simulink subsystem "h_bridge_v2"  (R2023a)
settings: Solver=VariableStepAuto  StartTime=0.0  StopTime=10.0  RelTol=1e-3
libraries: fl_lib x7, nesl_utility x4, dspstat3 x1
settings Model: Creator=motya  LastModifiedBy=motya

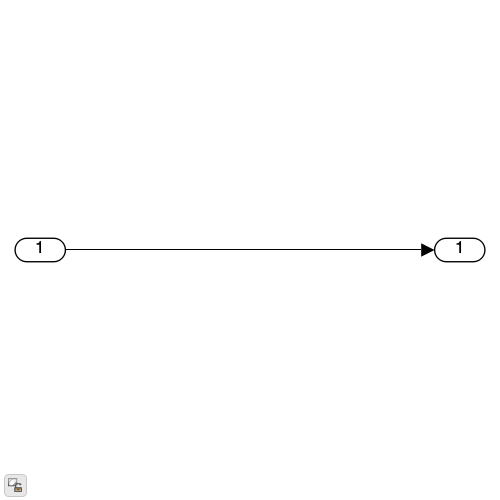
[thumbnail: Simulink's stored preview of the top-level diagram]
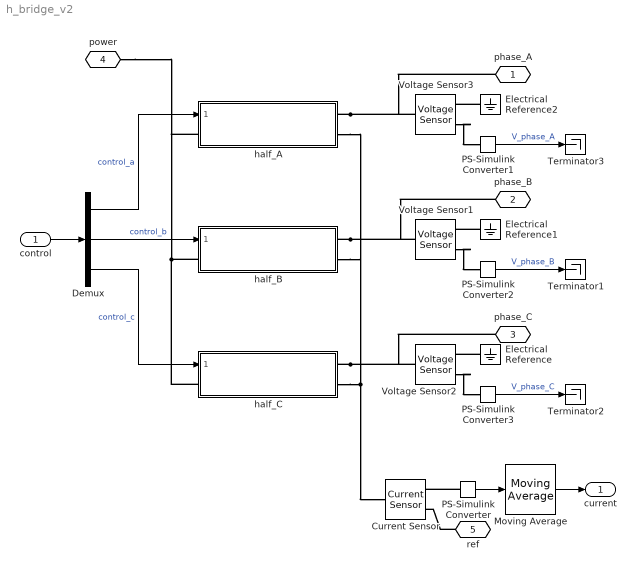
== system h_bridge_v2 ==
  control : Inport
  Current Sensor : fl_lib/Electrical/Electrical Sensors/Current Sensor
  Demux : Demux  Outputs=3
  Electrical Reference : fl_lib/Electrical/Electrical Elements/Electrical Reference
  Electrical Reference1 : fl_lib/Electrical/Electrical Elements/Electrical Reference
  Electrical Reference2 : fl_lib/Electrical/Electrical Elements/Electrical Reference
  Moving Average : dspstat3/Moving Average  Method=Sliding window  ForgettingFactorPort=off  SpecifyWindowLength=on  WindowLength=4  OverlapLength=3  AllowArbitraryInputLength=off  ForgettingFactor=0.9  SimulateUsing=Code generation
  PS-Simulink Converter{,1..3} (4 alike) : nesl_utility/PS-Simulink Converter  PhysicalDomain=network_engine_domain  SubClassName=ps_output  LeftPortType=input  RightPortType=output  PseudoPeriodic=off  Frequencies=[]  VectorFormat=inherit  Unit=inherit  AffineConversion=off
  Terminator1 : Terminator
  Terminator2 : Terminator
  Terminator3 : Terminator
  Voltage Sensor1 : fl_lib/Electrical/Electrical Sensors/Voltage Sensor
  Voltage Sensor2 : fl_lib/Electrical/Electrical Sensors/Voltage Sensor
  Voltage Sensor3 : fl_lib/Electrical/Electrical Sensors/Voltage Sensor
  half_A : Subsystem  ReferencedSubsystem=half_bridge_v2
  half_B : Subsystem  ReferencedSubsystem=half_bridge_v2
  half_C : Subsystem  ReferencedSubsystem=half_bridge_v2
  phase_A : PMIOPort  Side=Right
  phase_B : PMIOPort  Port=2  Side=Right
  phase_C : PMIOPort  Port=3  Side=Right
  power : PMIOPort  Port=4  Side=Left
  ref : PMIOPort  Port=5  Side=Right
  current : Outport
  wires:
  Demux/1 -> half_A/1  "control_a"
  Demux/2 -> half_B/1  "control_b"
  Demux/3 -> half_C/1  "control_c"
  Moving Average/1 -> current/1
  PS-Simulink Converter/1 -> Moving Average/1
  PS-Simulink Converter3/1 -> Terminator2/1  "V_phase_C"
  PS-Simulink Converter2/1 -> Terminator1/1  "V_phase_B"
  PS-Simulink Converter1/1 -> Terminator3/1  "V_phase_A"
  control/1 -> Demux/1
  connections:
  half_C/LConn1 -- half_A/LConn1 -- power/RConn1 -- half_B/LConn1
  half_C/RConn2 -- half_B/RConn2 -- half_A/RConn2 -- Current Sensor/LConn1
  half_A/RConn1 -- phase_A/RConn1 -- Voltage Sensor3/LConn1
  half_C/RConn1 -- Voltage Sensor2/LConn1 -- phase_C/RConn1
  half_B/RConn1 -- phase_B/RConn1 -- Voltage Sensor1/LConn1
  PS-Simulink Converter/LConn1 -- Current Sensor/RConn1
  ref/RConn1 -- Current Sensor/RConn2
  Voltage Sensor2/RConn1 -- PS-Simulink Converter3/LConn1
  Electrical Reference/LConn1 -- Voltage Sensor2/RConn2
  Voltage Sensor1/RConn1 -- PS-Simulink Converter2/LConn1
  Electrical Reference1/LConn1 -- Voltage Sensor1/RConn2
  Voltage Sensor3/RConn1 -- PS-Simulink Converter1/LConn1
  Electrical Reference2/LConn1 -- Voltage Sensor3/RConn2
